simulink model "SimMT"  (R2023b)
settings: Solver=VariableStepAuto  StartTime=0.0  StopTime=25  RelTol=1e-3
values from neighbouring files (symbols this model uses):
  b1 = 1000    [MT.m]    (also in SimulinkMT.m)
  k1 = 16182    [MT.m]    (also in SimulinkMT.m)
  k2 = 19000    [MT.m]    (also in SimulinkMT.m)
  m1 = 290    [MT.m]    (also in SimulinkMT.m)
  m2 = 59    [MT.m]    (also in SimulinkMT.m)

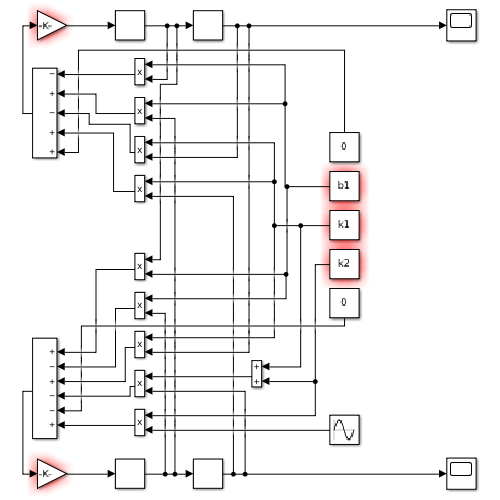
[thumbnail: Simulink's stored preview of the top-level diagram]
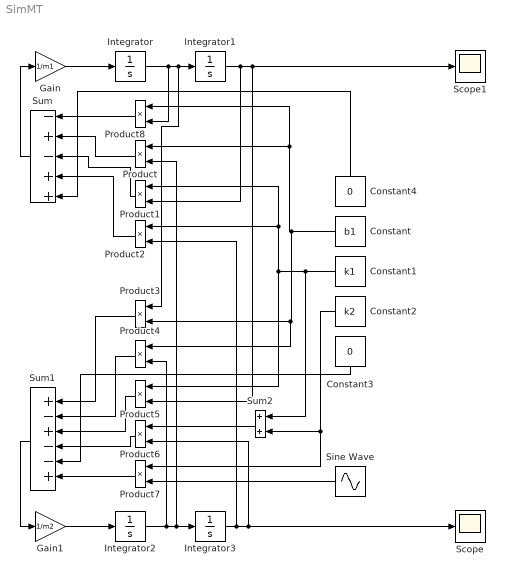
== system SimMT ==
  Constant : Constant  Value=b1
  Constant1 : Constant  Value=k1
  Constant2 : Constant  Value=k2
  Constant3 : Constant  Value=0
  Constant4 : Constant  Value=0
  Gain : Gain  Gain=1/m1
  Gain1 : Gain  Gain=1/m2
  Integrator{,1..3} (4 alike) : Integrator
  Product{,1..8} (9 alike) : Product
  Scope : Scope
  Scope1 : Scope
  Sine Wave : Sin  Amplitude=0.05  Frequency=0.5*pi  SampleTime=0
  Sum : Sum  Inputs=-+-++
  Sum1 : Sum  Inputs=+-+--+
  Sum2 : Sum
  wires:
  Integrator/1 -> Product8/2, Product3/1, Integrator1/1
  Integrator2/1 -> Product4/2, Product/2, Integrator3/1
  Gain1/1 -> Integrator2/1
  Gain/1 -> Integrator/1
  Product3/1 -> Sum1/1
  Product4/1 -> Sum1/2
  Product5/1 -> Sum1/3
  Product6/1 -> Sum1/4
  Product7/1 -> Sum1/6
  Integrator3/1 -> Product2/2, Product6/2, Scope/1
  Integrator1/1 -> Product1/2, Product5/2, Scope1/1
  Sum1/1 -> Gain1/1
  Sum/1 -> Gain/1
  Product8/1 -> Sum/1
  Product/1 -> Sum/2
  Product1/1 -> Sum/3
  Product2/1 -> Sum/4
  Constant/1 -> Product4/1, Product3/2, Product/1, Product8/1
  Constant1/1 -> Sum2/1, Product5/1, Product2/1, Product1/1
  Sum2/1 -> Product6/1
  Constant2/1 -> Product7/1, Sum2/2
  Constant3/1 -> Sum1/5
  Constant4/1 -> Sum/5
  Sine Wave/1 -> Product7/2
